simulink model "PMSM_dq_transform"  (R2024b)
settings: Solver=ode1be  StartTime=0.0  StopTime=6  FixedStep=0.001  RelTol=1e-3
undefined symbols (not defined in the file): B, Jr1, L_d1, L_q1, lambda_af1, p1, R_s1, Tc, U_N_1
libraries: spsabctodq0Lib x1, spsPermanentMagnetSynchronousMachineLib x1, simulink x1, spsThreePhaseProgrammableVoltageSourceLib x1, sps_lib x1
settings Model: Creator=menda  LastModifiedBy=menda

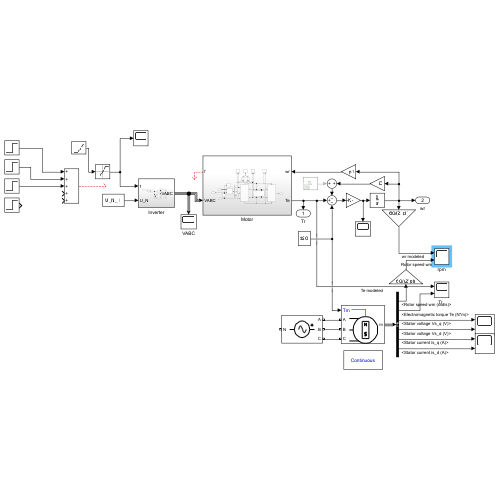
[thumbnail: Simulink's stored preview of the top-level diagram]
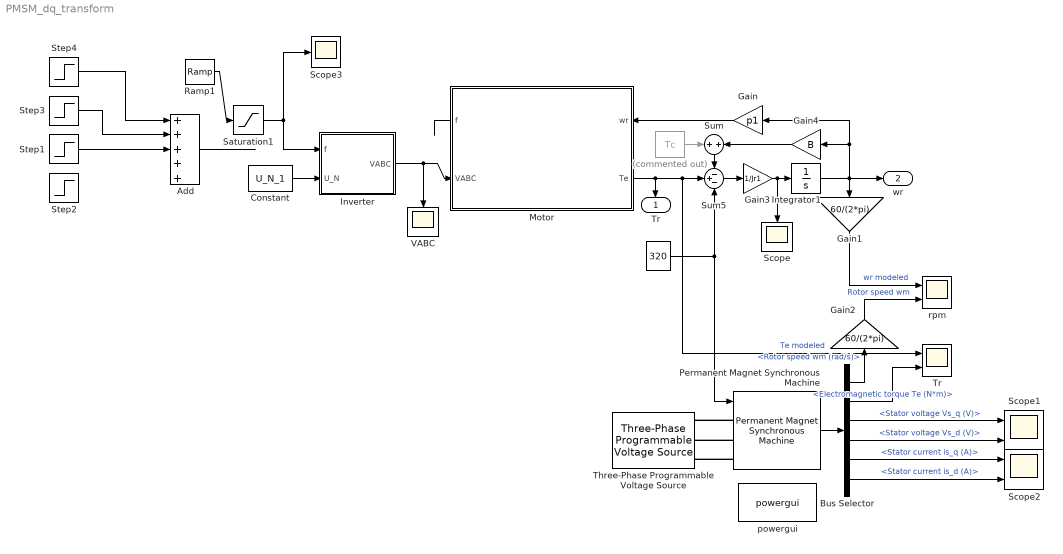
== system PMSM_dq_transform ==
  " " : Constant  Commented=on  Value=Tc
  "  " : Constant  Value=320
  Add : Sum  Inputs=+++++
  Bus Selector : BusSelector  OutputSignals=Rotor speed wm (rad/s),Electromagnetic torque Te (N*m),Stator voltage Vs_q (V),Stator voltage Vs_d (V),Stator current is_q (A),Stator current is_d (A)
  Constant : Constant  Value=U_N_1
  Gain : Gain  Gain=p1
  Gain1 : Gain  Gain=60/(2*pi)
  Gain2 : Gain  Gain=60/(2*pi)
  Gain3 : Gain  Gain=1/Jr1
  Gain4 : Gain  Gain=B
  Integrator1 : Integrator
  Inverter : Subsystem
  Motor : Subsystem
      settings: PortSchema="{\"entries\":[{\"content\":{\"sides\":[{\"content\":{\"connectorIds\":[\"Out2\",\"In1\"]},\"type\":\"ConnectorPlacement.EquallySpacedRectSide\",\"uuid\":\"b3ca4081-45ee-48b2-b21f-a1b8933fa16b\"},{\"content\":{\"connectorIds\":[\"In2\",\"Out1\"],\"side\":\"RIGHT\"},\"type\":\"ConnectorPlacement.EquallySpacedRectSide\",\"uuid\":\"10245e3e-2b38-411c-a0d3-68d04e2b29a2\"},{\"content\":{\"side\":\"TOP\"},\"type\":\"ConnectorPlacement.EquallySpacedRectSide\",\"uuid\":\"4010b917-fe94-424e-8ed8-75813c10a057\"}]},\"type\":\"ConnectorPlacement.EquallySpacedConnector\",\"uuid\":\"e5db9b22-11f2-430b-ab3a-b92abc903b6c\"}],\"packageUris\":[\"http://schema.mathworks.com/mf0/Connector/R2020b\"],\"version\":\"1.0\"}"
  Permanent Magnet Synchronous Machine : spsPermanentMagnetSynchronousMachineLib/Permanent Magnet Synchronous Machine  NbPhases=3  FluxDistribution=Sinusoidal  RotorType=Salient-pole  MechanicalLoad=Torque Tm  PresetModel=No  ShowDetailedParameters=on  MeasurementBus=off  Resistance=R_s1  Inductance=8.5e-3  dqInductances=[L_d1,L_q1]  La=0.000395  MachineConstant=Flux linkage established by magnets (V.s)  Flux=lambda_af1  VoltageCst=1000.1854  TorqueCst=8.2715  Flat=120  Mechanical=[Jr1 B p1 0]  PolePairs=4  InitialConditions=[0,0,0,0]  InitialConditions5ph=[0 0 0 0 0 0]  RefAngle=90 degrees behind phase A axis (modified Park)  IterativeDiscreteModel=Trapezoidal non iterative  TsBlock=-1  TsPowergui=0
  Ramp1 : simulink/Sources/Ramp  slope=100  start=0  InitialOutput=0
  Saturation1 : Saturate  UpperLimit=100
  Scope : Scope
  Scope1 : Scope  NumInputPorts=2
  Scope2 : Scope  NumInputPorts=2
  Scope3 : Scope
  Step1 : Step  Time=2  After=20  SampleTime=0
  Step2 : Step  After=20  SampleTime=0
  Step3 : Step  After=20  SampleTime=0
  Step4 : Step  Time=0  After=20  SampleTime=0
  Sum : Sum  Inputs=+|+
  Sum5 : Sum  Inputs=-+-
  Three-Phase Programmable Voltage Source : spsThreePhaseProgrammableVoltageSourceLib/Three-Phase Programmable Voltage Source  PositiveSequence="[U_N_1  0 20]"  VariationEntity=None  VariationType=Table of time-amplitude pairs  VariationTypeAlt=Step  VariationStep=0.5  VariationRate=10  VariationMagnitude=0.3  VariationFrequency=2  VariationTiming=[1 2]  VariationPhaseA=off  Amplitudes=[1 0.8 1.2 1.0]  TimeValues=[0 0.1 0.15 0.2]  HarmonicGeneration=off  HarmonicA=[3 0.2 -25 0]  HarmonicB=[2 0.15 35 2]  Timing="[0.05  3]"  BusType=swing  Pref=0  Qref=0  Qmin=-inf  Qmax=inf
  "Tr  " : Scope  NumInputPorts=2
  VABC : Scope
  powergui : sps_lib/powergui  Priority=1  SimulationMode=Continuous  SampleTime=50e-6  frequency=60  Iterations=50  frequencyindice=0  Pbase=100e6  ErrMax=1e-4  UnitsV=kV  UnitsW=MW  buscounter=0  FunctionMessages=off  echomessages=off  EnableUseOfTLC=off  CurrentSourceSwitches=off  DisableSnubberDevices=off  DisableRonSwitches=off  DisableVfSwitches=off  DisplayEquations=off  AutomaticDiscreteSolvers=off  SolverType=Tustin/Backward Euler (TBE)  Interpol=off  ExternalGateDelay=off  methode=off  Ts=100  x0status=blocks  SPID=on  SwTol=0  HookPort=off  NonlinearTolerance=1e-4  nMaxIteration=100  ContinueOnMaxIteration=off  RestoreLinks=warning  ResistiveCurrentMeasurement=off  Frange=[0:2:500]  Ylog=off  Xlog=on  ShowGrid=off  save=off  variable=ZData  structure=0  ZoomFFT=off  StartTime=0.0  cycles=1  DisplayStyle=1  fundamental=60  FreqAxis=off  MaxFrequency=1000  frequencyindicesteady=1  RmsSteady=1  display=off
  rpm : Scope  NumInputPorts=2
  Tr : Outport
  wr : Outport  Port=2
  wires:
  Gain4/1 -> Sum/2
  Gain3/1 -> Scope/1, Integrator1/1
  Integrator1/1 -> wr/1, Gain1/1, Gain4/1, Gain/1
  Motor/1(Te) -> Sum5/2, "Tr  "/1, Tr/1  "Te modeled"
  "  "/1 -> Permanent Magnet Synchronous Machine/1, Sum5/3
  Sum5/1 -> Gain3/1
  Gain/1 -> Motor/2(wr)
  Sum/1 -> Sum5/1
  " "/1 -> Sum/1
  Gain1/1 -> rpm/1  "wr modeled"
  Inverter/1(VABC) -> Motor/1(VABC), VABC/1
  Permanent Magnet Synchronous Machine/1 -> Bus Selector/1
  Bus Selector/1 -> Gain2/1  "<Rotor speed wm (rad/s)>"
  Bus Selector/2 -> "Tr  "/2  "<Electromagnetic torque Te (N*m)>"
  Gain2/1 -> rpm/2  "Rotor speed wm"
  Bus Selector/3 -> Scope1/1  "<Stator voltage Vs_q (V)>"
  Bus Selector/4 -> Scope1/2  "<Stator voltage Vs_d (V)>"
  Bus Selector/5 -> Scope2/1  "<Stator current is_q (A)>"
  Bus Selector/6 -> Scope2/2  "<Stator current is_d (A)>"
  Ramp1/1 -> Saturation1/1
  Motor/2(f) -> ?
  Add/1 -> ?
  Step4/1 -> Add/1
  Step3/1 -> Add/2
  Constant/1 -> Inverter/2(U_N)
  Step1/1 -> Add/3
  Saturation1/1 -> Scope3/1, Inverter/1(f)
  connections:
  Permanent Magnet Synchronous Machine/LConn1 -- Three-Phase Programmable Voltage Source/RConn1
  Permanent Magnet Synchronous Machine/LConn2 -- Three-Phase Programmable Voltage Source/RConn2
  Permanent Magnet Synchronous Machine/LConn3 -- Three-Phase Programmable Voltage Source/RConn3

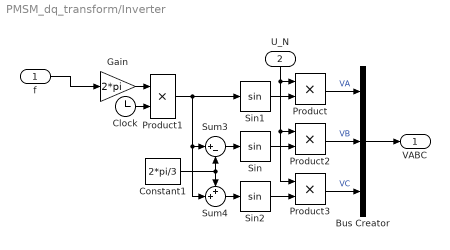
== system PMSM_dq_transform/Inverter ==
  f : Inport
  U_N : Inport  Port=2
  Bus Creator : BusCreator  Inputs=3
  Clock : Clock
      settings: Decimation=100
  Constant1 : Constant  Value=2*pi/3
  Gain : Gain  Gain=2*pi
  Product{,1..3} (4 alike) : Product
  Sin : Trigonometry
  Sin1 : Trigonometry
  Sin2 : Trigonometry
  Sum3 : Sum  Inputs=|+-
  Sum4 : Sum  Inputs=++|
  VABC : Outport
  wires:
  Product1/1 -> Sum3/1, Sum4/2, Sin1/1
  Sin/1 -> Product2/2
  U_N/1 -> Product3/1, Product2/1, Product/1
  Sum4/1 -> Sin2/1
  Sin2/1 -> Product3/2
  Sin1/1 -> Product/2
  Sum3/1 -> Sin/1
  Constant1/1 -> Sum4/1, Sum3/2
  Product/1 -> Bus Creator/1  "VA"
  Product3/1 -> Bus Creator/3  "VC"
  Product2/1 -> Bus Creator/2  "VB"
  Gain/1 -> Product1/1
  Bus Creator/1 -> VABC/1
  Clock/1 -> Product1/2
  f/1 -> Gain/1

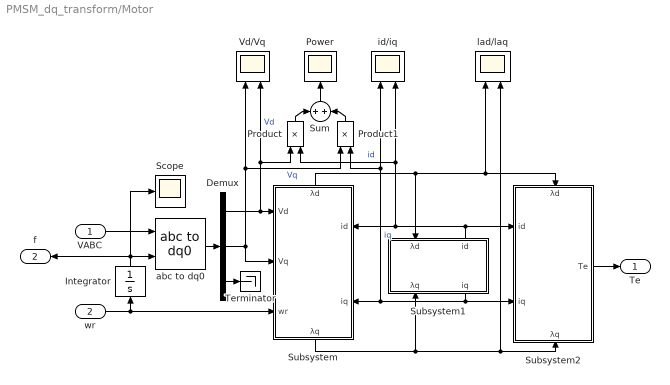
== system PMSM_dq_transform/Motor ==
  VABC : Inport
  wr : Inport  Port=2
  Demux : Demux  Outputs=3
  Integrator : Integrator
  Power : Scope
  Product : Product
  Product1 : Product
  Scope : Scope
  Subsystem : Subsystem
      settings: PortSchema="{\"entries\":[{\"content\":{\"sides\":[{\"content\":{\"connectorIds\":[\"In1\",\"In2\",\"In3\"]},\"type\":\"ConnectorPlacement.EquallySpacedRectSide\",\"uuid\":\"3302189e-c65f-4fe9-82d9-6d0de0f94bf0\"},{\"content\":{\"connectorIds\":[\"In4\",\"In5\"],\"side\":\"RIGHT\"},\"type\":\"ConnectorPlacement.EquallySpacedRectSide\",\"uuid\":\"6cab5dbb-df1e-4dcd-9af1-89a25abd4563\"},{\"content\":{\"connectorIds\":[\"Out2\"],\"side\":\"TOP\"},\"type\":\"ConnectorPlacement.EquallySpacedRectSide\",\"uuid\":\"08bda315-91a6-4f85-83b2-9931e6491f66\"},{\"content\":{\"connectorIds\":[\"Out1\"],\"side\":\"BOTTOM\"},\"type\":\"ConnectorPlacement.EquallySpacedRectSide\",\"uuid\":\"3edf6519-f00a-4956-811f-61f08f5f6888\"}]},\"type\":\"ConnectorPlacement.EquallySpacedConnector\",\"uuid\":\"ed3de687-0b42-4981-aea3-2b088fe6e133\"}],\"packageUris\":[\"http://schema.mathworks.com/mf0/Connector/R2020b\"],\"version\":\"1.0\"}"
  Subsystem1 : Subsystem
      settings: PortSchema="{\"entries\":[{\"content\":{\"sides\":[{\"content\":{},\"type\":\"ConnectorPlacement.EquallySpacedRectSide\",\"uuid\":\"c851675a-9655-496b-b707-efae19577f68\"},{\"content\":{\"side\":\"RIGHT\"},\"type\":\"ConnectorPlacement.EquallySpacedRectSide\",\"uuid\":\"54f56f5f-62b7-4f63-be33-084e502ccd16\"},{\"content\":{\"connectorIds\":[\"In1\",\"Out2\"],\"side\":\"TOP\"},\"type\":\"ConnectorPlacement.EquallySpacedRectSide\",\"uuid\":\"4fa1fd5e-d680-48b2-b970-595469dd5531\"},{\"content\":{\"connectorIds\":[\"In2\",\"Out1\"],\"side\":\"BOTTOM\"},\"type\":\"ConnectorPlacement.EquallySpacedRectSide\",\"uuid\":\"6f710f49-7fb9-4c82-8050-8f64bc190e29\"}]},\"type\":\"ConnectorPlacement.EquallySpacedConnector\",\"uuid\":\"59c03cd4-7e68-485c-a3a6-ec57c6e65b02\"}],\"packageUris\":[\"http://schema.mathworks.com/mf0/Connector/R2020b\"],\"version\":\"1.0\"}"
  Subsystem2 : Subsystem
      settings: PortSchema="{\"entries\":[{\"content\":{\"sides\":[{\"content\":{\"connectorIds\":[\"In1\",\"In2\"]},\"type\":\"ConnectorPlacement.EquallySpacedRectSide\",\"uuid\":\"b3ca4081-45ee-48b2-b21f-a1b8933fa16b\"},{\"content\":{\"connectorIds\":[\"Out1\"],\"side\":\"RIGHT\"},\"type\":\"ConnectorPlacement.EquallySpacedRectSide\",\"uuid\":\"10245e3e-2b38-411c-a0d3-68d04e2b29a2\"},{\"content\":{\"connectorIds\":[\"In3\"],\"side\":\"TOP\"},\"type\":\"ConnectorPlacement.EquallySpacedRectSide\",\"uuid\":\"4010b917-fe94-424e-8ed8-75813c10a057\"},{\"content\":{\"connectorIds\":[\"In4\"],\"side\":\"BOTTOM\"},\"type\":\"ConnectorPlacement.EquallySpacedRectSide\",\"uuid\":\"f86bf731-613b-408f-8484-c12c8c456b3b\"}]},\"type\":\"ConnectorPlacement.EquallySpacedConnector\",\"uuid\":\"e5db9b22-11f2-430b-ab3a-b92abc903b6c\"}],\"packageUris\":[\"http://schema.mathworks.com/mf0/Connector/R2020b\"],\"version\":\"1.0\"}"
  Sum : Sum  Inputs=+|+
  Terminator : Terminator
  Vd/Vq : Scope  NumInputPorts=2
  abc to dq0 : spsabctodq0Lib/abc to dq0  Alignment=Aligned with phase A axis
  id/iq : Scope  NumInputPorts=2
  lad/laq : Scope  NumInputPorts=2
  Te : Outport
  f : Outport  Port=2
  wires:
  VABC/1 -> abc to dq0/1
  wr/1 -> Subsystem/3(wr), Integrator/1
  Integrator/1 -> f/1, Scope/1, abc to dq0/2
  abc to dq0/1 -> Demux/1
  Demux/3 -> Terminator/1
  Subsystem1/2(id) -> Subsystem/4(id), Product/2, id/iq/2, Subsystem2/1(id)  "id"
  Subsystem/2(λd) -> lad/laq/1, Subsystem2/3(λd), Subsystem1/1(λd)
  Subsystem/1(λq) -> Subsystem2/4(λq), lad/laq/2, Subsystem1/2(λq)
  Subsystem1/1(iq) -> Subsystem/5(iq), Product1/2, id/iq/1, Subsystem2/2(iq)  "iq"
  Subsystem2/1(Te) -> Te/1
  Demux/2 -> Subsystem/2(Vq), Vd/Vq/1, Product1/1  "Vq"
  Demux/1 -> Subsystem/1(Vd), Vd/Vq/2, Product/1  "Vd"
  Product/1 -> Sum/1
  Sum/1 -> Power/1
  Product1/1 -> Sum/2

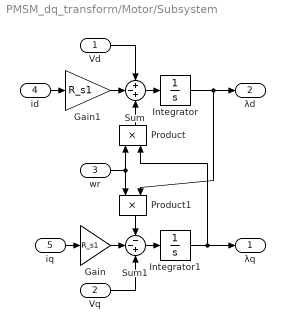
== system PMSM_dq_transform/Motor/Subsystem ==
  Vd : Inport
  Vq : Inport  Port=2
  wr : Inport  Port=3
  id : Inport  Port=4
  iq : Inport  Port=5
  Gain : Gain  Gain=R_s1
  Gain1 : Gain  Gain=R_s1
  Integrator : Integrator
  Integrator1 : Integrator
  Product : Product
  Product1 : Product
  Sum : Sum  Inputs=+-+
  Sum1 : Sum  Inputs=--+
  λq : Outport
  λd : Outport  Port=2
  wires:
  Vd/1 -> Sum/1
  Vq/1 -> Sum1/3
  Product/1 -> Sum/3
  Product1/1 -> Sum1/1
  Sum/1 -> Integrator/1
  Integrator/1 -> λd/1, Product1/2
  Sum1/1 -> Integrator1/1
  Integrator1/1 -> λq/1, Product/2
  wr/1 -> Product/1, Product1/1
  iq/1 -> Gain/1
  Gain/1 -> Sum1/2
  Gain1/1 -> Sum/2
  id/1 -> Gain1/1

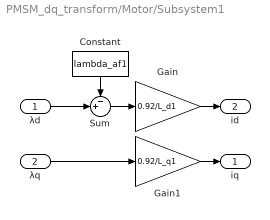
== system PMSM_dq_transform/Motor/Subsystem1 ==
  λd : Inport
  λq : Inport  Port=2
  Constant : Constant  Value=lambda_af1
  Gain : Gain  Gain=0.92/L_d1
  Gain1 : Gain  Gain=0.92/L_q1
  Sum : Sum  Inputs=-+|
  iq : Outport
  id : Outport  Port=2
  wires:
  λd/1 -> Sum/2
  Constant/1 -> Sum/1
  Sum/1 -> Gain/1
  Gain/1 -> id/1
  λq/1 -> Gain1/1
  Gain1/1 -> iq/1

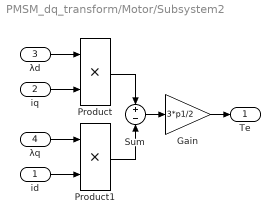
== system PMSM_dq_transform/Motor/Subsystem2 ==
  id : Inport
  iq : Inport  Port=2
  λd : Inport  Port=3
  λq : Inport  Port=4
  Gain : Gain  Gain=3*p1/2
  Product : Product
  Product1 : Product
  Sum : Sum  Inputs=+|-
  Te : Outport
  wires:
  λd/1 -> Product/1
  λq/1 -> Product1/1
  id/1 -> Product1/2
  iq/1 -> Product/2
  Product/1 -> Sum/1
  Product1/1 -> Sum/2
  Sum/1 -> Gain/1
  Gain/1 -> Te/1
